simulink model "PEMFuelCellSystem_Cathode_cEGR_SelfHumidifying_v01"  (R2025b)
settings: Solver=VariableStepAuto  StartTime=0.0  StopTime=100  MaxStep=0.1  RelTol=1e-3  AbsTol=1e-3
model workspace (MAT data in the model file):
  Gas_properties_block = 'PEMFuelCellSystem_Before_v01/Anode_Hydrogen_BOP/Gas Mixture
Properties'
  Gas_properties_candidates : object (value not decoded)
  T_TLU = [223.15 228.15 233.15 238.15 243.15 248.15 253.15 258.15 263.15 268.15 272.66 273.15 ... (115 elements, 1x115)]
  air_control_min_current_A = 3.8
  anode_separator_D = 0.02
  anode_separator_T0 = 20
  anode_separator_area = 0.000314159265359
  anode_separator_dp_nominal = 0.0005
  anode_separator_extra_length = 0.04
  anode_separator_laminar_fraction = 0.001
  anode_separator_length = 0.12
  anode_separator_mdot_nominal = 0.01
  anode_separator_p0 = 0.101325
  anode_separator_roughness = 1.5e-05
  anode_tube_D = 0.02
  cathode_channel_dp_nominal_MPa = 0.0368422
  cathode_channel_flow_area_m2 = 0.00403764556423
  cathode_channel_mdot_nominal_kg_s = 0.27182
  cathode_outlet_chamber_V = 0.2
  cathode_separator_D = 0.05
  cathode_separator_T0 = 20
  cathode_separator_area = 0.00407150407905
  cathode_separator_dp_nominal = 0.002
  cathode_separator_extra_length = 0.05
  cathode_separator_laminar_fraction = 0.001
  cathode_separator_length = 0.15
  cathode_separator_mdot_nominal = 0.40798
  cathode_separator_p0 = 0.101325
  cathode_separator_roughness = 1.5e-05
  cathode_tube_D = 0.05
  cegr_comp_map_t_denom_epsilon = 1e-09
  cegr_cond_tau = 1
  cegr_inlet_mixer_p0 = 0.101325
  cegr_outlet_chamber_p0 = 0.101325
  cegr_pipe_D = 0.072
  cegr_pipe_area = 0.00407150407905
  cegr_pipe_extra_length = 0.1
  cegr_pipe_length = 0.5
  cegr_pipe_p0 = 0.101325
  cegr_pipe_roughness = 1.5e-05
  cegr_valve_max_area = 0.001
  cegr_valve_open_min_area = 1e-10
  common_bp_valve_max_area = 0.00134
  common_bp_valve_open_min_area = 1e-10
  comp_inlet_mixer_V = 0.1
  comp_mdot_corr_TLU = [0 0 0 0 0 0.28 0.26 0.24 0.22 0.2 0.56 0.52 ... (15 elements, 5x3)]
  comp_p_ratio_TLU = [1 1.5 2 2.5 3]
  comp_rpm_TLU = [0 50000 80000]
  coolant_num_layers = 20
  coolant_num_passes = 12
  coolant_tube_D = 0.05
  coolant_w_channels = 1
  drive_cycle_current = [0 0 100 100]
  drive_cycle_power = [0 0 40 40]
  drive_cycle_time = [0 0.5 60.5 600]
  drive_cycle_voltage = [427.6 427.6 410 410]
  env_RH = 0.5
  env_T = 20
  env_p = 0.101325
  env_pSat_H2O = 0.00233931818334
  env_yH20 = 0.0115436377169
  env_yO2 = 0.21
  focused_anode_boundary_T_C = 20
  focused_anode_feed_p_MPa_abs = 0.3
  focused_anode_inlet_mdot_kg_s = 0.008
  focused_anode_inlet_p_MPa_abs = 0.161325
  focused_anode_outlet_p_MPa_abs = 0.101325
  focused_anode_pipe_area = 0.00246300864041
  focused_anode_pipe_extra_length = 0.1
  focused_anode_pipe_length = 1
  focused_anode_pipe_roughness = 1.5e-05
  focused_anode_yH2 = 0.9997
  focused_stack_temperature_C = 80
  humidifier_bypass_mode : string (value not decoded)
  intercooler_Dh = 0.05
  intercooler_T0 = 20
  intercooler_area = 0.00785398163397
  intercooler_cond_tau = 1
  intercooler_dp_nominal = 0.005
  intercooler_extra_length = 0.05
  intercooler_laminar_fraction = 0.001
  intercooler_length = 0.25
  intercooler_mdot_nominal = 0.40798
  intercooler_p0 = 0.101325
  intercooler_roughness = 1.5e-05
  pSat_H2O_TLU = [0.0039376926592 0.00720321689378 0.0128411282011 0.0223441068076 0.0380050105363 0.0632733889962 0.103238678713 0.165273175188 0.259872929049 0.401739659013 0.586936061043 0.611151401419 ... (115 elements, 1x115)]
  pSat_TLU = [3379.45709837 5023.40410987 1277.63968517 0.0039376926592 3379.45809837 5023.40510987 1277.64068517 0.00720321689378 3379.45909837 5023.40610987 1277.64168517 0.0128411282011 ... (460 elements, 4x115)]
  radiator_H = 0.5
  radiator_L = 1
  radiator_N_fins = 12000
  radiator_N_tubes = 25
  radiator_W = 0.025
  radiator_air_area_fins = 11.5625
  radiator_air_area_primary = 1.223125
  radiator_cp = 910
  radiator_eta_fin = 0.7
  radiator_fin_spacing = 0.002
  radiator_gap_H = 0.0192708333333
  radiator_rho = 2700
  radiator_t_wall = 0.0001
  radiator_tube_H = 0.0015
  radiator_tube_Leq = 2.5
  routeA_air_control_mode_id = 2
  routeA_air_pid_Ki = 0.5
  routeA_air_pid_Kp = 5
  routeA_anode_inlet_pressure_MPa_abs = 0.161325
  routeA_anode_purge_enable = 1
  routeA_anode_purge_off_n2_mole_fraction = 0.1
  routeA_anode_purge_on_n2_mole_fraction = 0.5
  routeA_anode_recirculation_base_command = 0.2
  routeA_anode_recirculation_current_gain_A_inv = 0.00204081632653
  routeA_anode_rh_setpoint = 1
  routeA_backpressure_control_mode_id = 1
  routeA_cathode_humidifier_gain = 1
  routeA_cathode_rh_setpoint = 1
  routeA_cegr_enabled = 1
  routeA_cegr_valve_mode_id = 1
  routeA_command_profile = [0 0.5 60.5 600 0.101325 0.101325 0.101325 0.101325 20 20 20 20 ... (92 elements, 4x23)]
  routeA_command_profile_baseline = [0.101325 20 0.21 0.0115436377169 0.045 3 0.5 0.1613 1 1 0 70 ... (22 elements, 1x22)]
  routeA_command_profile_fields : string (value not decoded)
  routeA_command_profile_schema : string (value not decoded)
  routeA_current_default_ref_A = 28
  routeA_egr_control_Ki_area = 3.92699081699e-05
  routeA_egr_control_Kp_area = 0.000196349540849
  routeA_egr_control_mode_id = 1
  routeA_egr_target_input_mode_id = 1
  routeA_egr_valve_actuator_tau = 0.5
  routeA_egr_valve_area_direct = 3.92699081699e-06
  routeA_external_case_enabled = 0
  routeA_parameter_layer : string (value not decoded)
  routeA_stack_temperature_set_C = 80
  routeA_target_egr_ratio_comp_in = 0.02
  routeA_voltage_current_max_A = 392
  routeA_voltage_current_min_A = 0
  routeA_voltage_default_ref_V = 394.9
  routeA_voltage_pi_Ki = 0.05
  routeA_voltage_pi_Kp = 1
  separator_condensation_enabled = 1
  separator_l2_efficiency = 0.5
  separator_l2_source : string (value not decoded)
  stack_alpha = 0.7
  stack_area = 380
  stack_iL = 2.5
  stack_io = 0.0001
  stack_mea_cp = 870
  stack_mea_rho = 1800
  stack_num_cells = 606
  stack_num_channels = 8
  stack_t_gdl = 250
  stack_t_membrane = 125
  stack_w_channels = 1.16496474502
  tank_T = 20
  tank_V = 120
  tank_p = 70
  tank_yH2 = 0.9997
libraries: FuelCell_lib x44, nesl_utility x32, fl_lib x32, slpidlib x4
(part 2 of 4)

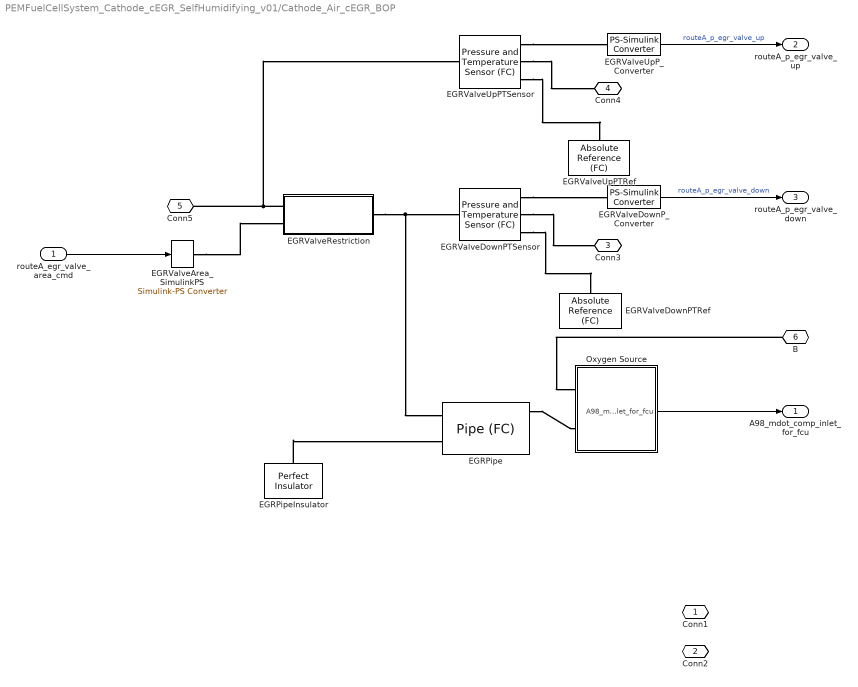
== system PEMFuelCellSystem_Cathode_cEGR_SelfHumidifying_v01/Cathode_Air_cEGR_BOP ==
  routeA_egr_valve_area_cmd : Inport
  EGRPipe : FuelCell_lib/elements/Pipe (FC)  length=cegr_pipe_length m  area=cegr_pipe_area m^2  Dh=cegr_pipe_D m  extra_length=cegr_pipe_extra_length m  roughness=cegr_pipe_roughness m  Re_lam=2000  Re_tur=4000  shape_factor=64  Nu_lam=3.66  tau_c=cegr_cond_tau s  isCond=[0; 0; 0; 1]  volMeas=false  compMeas=FuelCell.enum.Composition.Mole  p0=cegr_pipe_p0 MPa  T0=env_T degC  comp=FuelCell.enum.Composition.Mole  y0=[1-env_yO2-env_yH20; env_yO2; 0; env_yH20]  x0=[1-env_yO2-env_yH20; env_yO2; 0; env_yH20]
      settings: InternalSimscapePortConfiguration="{\"Bottom\":[{\"id\":\"MIn\",\"label\":\"M_in\",\"type\":\"input\"},{\"id\":\"TIn\",\"label\":\"T_in\",\"type\":\"input\"}],\"Left\":[{\"id\":\"A\",\"label\":\"A\",\"type\":\"FuelCell.FuelCell\"},{\"id\":\"H\",\"label\":\"H\",\"type\":\"foundation.thermal.thermal\"}],\"Right\":[{\"id\":\"B\",\"label\":\"B\",\"type\":\"FuelCell.FuelCell\"}],\"Top\":[]}"
  EGRPipeInsulator : fl_lib/Thermal/Thermal Elements/Perfect Insulator  T_specify=off  T_priority=None  T=env_T degC  T_nominal_specify=off  T_nominal_value=1  T_nominal_unit=K
  EGRValveArea_SimulinkPS : nesl_utility/Simulink-PS Converter  PhysicalDomain=network_engine_domain  SubClassName=ps_input  LeftPortType=input  RightPortType=output  PseudoPeriodic=off  Frequencies=[]  NoiseDistribution=none  NoiseParameters=[]  Unit=m^2  AffineConversion=off  FilteringAndDerivatives=provide  SimscapeFilterOrder=1  InputFilterTimeConstant=0.001  UdotUserProvided=0
  EGRValveDownPTRef : FuelCell_lib/elements/Absolute Reference (FC)
      settings: InternalSimscapePortConfiguration="{\"Bottom\":[],\"Left\":[{\"id\":\"A\",\"label\":\"\",\"type\":\"FuelCell.FuelCell\"}],\"Right\":[],\"Top\":[]}"
  EGRValveDownPTSensor : FuelCell_lib/sensors/Pressure and Temperature Sensor (FC)
      settings: InternalSimscapePortConfiguration="{\"Bottom\":[],\"Left\":[{\"id\":\"A\",\"label\":\"A\",\"type\":\"FuelCell.FuelCell\"}],\"Right\":[{\"id\":\"P\",\"label\":\"P\",\"type\":\"output\"},{\"id\":\"T\",\"label\":\"T\",\"type\":\"output\"},{\"id\":\"B\",\"label\":\"B\",\"type\":\"FuelCell.FuelCell\"}],\"Top\":[]}"
  EGRValveDownP_Converter : nesl_utility/PS-Simulink Converter  PhysicalDomain=network_engine_domain  SubClassName=ps_output  LeftPortType=input  RightPortType=output  PseudoPeriodic=off  Frequencies=[]  VectorFormat=inherit  Unit=inherit  AffineConversion=off
  EGRValveRestriction : Subsystem  Variant=on
  EGRValveUpPTRef : FuelCell_lib/elements/Absolute Reference (FC)
      settings: InternalSimscapePortConfiguration="{\"Bottom\":[],\"Left\":[{\"id\":\"A\",\"label\":\"\",\"type\":\"FuelCell.FuelCell\"}],\"Right\":[],\"Top\":[]}"
  EGRValveUpPTSensor : FuelCell_lib/sensors/Pressure and Temperature Sensor (FC)
      settings: InternalSimscapePortConfiguration="{\"Bottom\":[],\"Left\":[{\"id\":\"A\",\"label\":\"A\",\"type\":\"FuelCell.FuelCell\"}],\"Right\":[{\"id\":\"P\",\"label\":\"P\",\"type\":\"output\"},{\"id\":\"T\",\"label\":\"T\",\"type\":\"output\"},{\"id\":\"B\",\"label\":\"B\",\"type\":\"FuelCell.FuelCell\"}],\"Top\":[]}"
  EGRValveUpP_Converter : nesl_utility/PS-Simulink Converter  PhysicalDomain=network_engine_domain  SubClassName=ps_output  LeftPortType=input  RightPortType=output  PseudoPeriodic=off  Frequencies=[]  VectorFormat=inherit  Unit=inherit  AffineConversion=off
  Oxygen Source : Subsystem  Tag=PublishSubsystem
      mask Display:
      | plot(0, 0)
      | plot(100, 100)
      | 
      | n = 80;
      | r1 = 15;
      | r2 = 30;
      | 
      | plot(cos(linspace(0, 2*pi, n))*r1 + 65, sin(linspace(0, 2*pi, n))*r1 + 50)
      | plot(cos(linspace(0, 2*pi, n))*r2 + 65, sin(linspace(0, 2*pi, n))*r2 + 50)
      | 
      | plot([65 30 30 42], [80 80 70 70])
  Conn1 : PMIOPort  Side=Right
  Conn2 : PMIOPort  Port=2  Side=Right
  Conn3 : PMIOPort  Port=3  Side=Right
  Conn4 : PMIOPort  Port=4  Side=Right
  Conn5 : PMIOPort  Port=5  Side=Left
  B : PMIOPort  Port=6  Side=Left
  A98_mdot_comp_inlet_for_fcu : Outport
  routeA_p_egr_valve_up : Outport  Port=2
  routeA_p_egr_valve_down : Outport  Port=3
  wires:
  routeA_egr_valve_area_cmd/1 -> EGRValveArea_SimulinkPS/1
  EGRValveUpP_Converter/1 -> routeA_p_egr_valve_up/1  "routeA_p_egr_valve_up"
  EGRValveDownP_Converter/1 -> routeA_p_egr_valve_down/1  "routeA_p_egr_valve_down"
  Oxygen Source/1(A98_mdot_comp_inlet_for_fcu) -> A98_mdot_comp_inlet_for_fcu/1
  connections:
  EGRValveUpPTSensor/RConn2 -- Conn4/RConn1
  EGRValveUpPTSensor/RConn1 -- EGRValveUpP_Converter/LConn1
  EGRValveArea_SimulinkPS/RConn1 -- EGRValveRestriction/LConn2
  EGRValveRestriction/LConn1 -- Conn5/RConn1 -- EGRValveUpPTSensor/LConn1
  EGRValveRestriction/RConn1 -- EGRPipe/LConn1 -- EGRValveDownPTSensor/LConn1
  EGRPipeInsulator/LConn1 -- EGRPipe/LConn2
  EGRPipe/RConn1 -- Oxygen Source/LConn2
  EGRValveUpPTSensor/RConn3 -- EGRValveUpPTRef/LConn1
  EGRValveDownPTSensor/RConn1 -- EGRValveDownP_Converter/LConn1
  EGRValveDownPTSensor/RConn2 -- Conn3/RConn1
  EGRValveDownPTSensor/RConn3 -- EGRValveDownPTRef/LConn1
  B/RConn1 -- Oxygen Source/LConn1

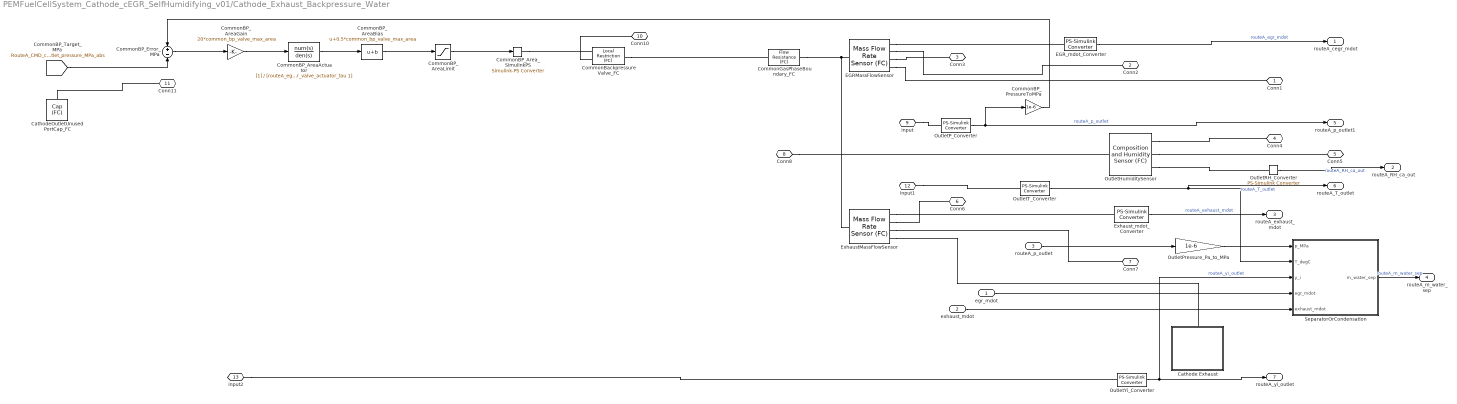
== system PEMFuelCellSystem_Cathode_cEGR_SelfHumidifying_v01/Cathode_Exhaust_Backpressure_Water ==
  egr_mdot : Inport
  exhaust_mdot : Inport  Port=2
  routeA_p_outlet : Inport  Port=3
  Cathode Exhaust : Subsystem  Tag=PublishSubsystem
      settings: PortSchema="{\"entries\":[{\"content\":{\"sides\":[{\"content\":{\"connectorIds\":[]},\"type\":\"ConnectorPlacement.EquallySpacedRectSide\",\"uuid\":\"6344d1cf-22ea-4a51-9588-07afca0fac15\"},{\"content\":{\"connectorIds\":[],\"side\":\"RIGHT\"},\"type\":\"ConnectorPlacement.EquallySpacedRectSide\",\"uuid\":\"a3908f81-9410-4056-87cd-9faba76d3fb8\"},{\"content\":{\"connectorIds\":[\"LConn1\"],\"side\":\"TOP\"},\"type\":\"ConnectorPlacement.EquallySpacedRectSide\",\"uuid\":\"a1c9e24d-adb9-4361-8e9b-feafccbbdb81\"}]},\"type\":\"ConnectorPlacement.EquallySpacedConnector\",\"uuid\":\"d5180d8f-18a0-491d-9fff-909db43c9aea\"}],\"packageUris\":[\"http://schema.mathworks.com/mf0/Connector/R2020b\"],\"version\":\"1.0\"}"
  CathodeOutletUnusedPortCap_FC : FuelCell_lib/elements/Cap (FC)  p_specify=off  p_priority=None  p=101325 Pa  p_nominal_specify=off  p_nominal_value=1  p_nominal_unit=Pa  x_i_specify=off  x_i_priority=None  x_i=[1; 0; 0; 0]  x_i_nominal_specify=off  x_i_nominal_value=1  x_i_nominal_unit=1  T_specify=off  T_priority=None  T=293.15 K  T_nominal_specify=off  T_nominal_value=1  T_nominal_unit=K
      settings: InternalSimscapePortConfiguration="{\"Bottom\":[],\"Left\":[{\"id\":\"A\",\"label\":\"A\",\"type\":\"FuelCell.FuelCell\"}],\"Right\":[],\"Top\":[]}"
  CommonBP_AreaActuator : TransferFcn  Denominator=[routeA_egr_valve_actuator_tau 1]
  CommonBP_AreaBias : Bias  Bias=0.5*common_bp_valve_max_area
  CommonBP_AreaGain : Gain  Gain=20*common_bp_valve_max_area
  CommonBP_AreaLimit : Saturate  UpperLimit=common_bp_valve_max_area  LowerLimit=common_bp_valve_open_min_area
  CommonBP_Area_SimulinkPS : nesl_utility/Simulink-PS Converter  PhysicalDomain=network_engine_domain  SubClassName=ps_input  LeftPortType=input  RightPortType=output  PseudoPeriodic=off  Frequencies=[]  NoiseDistribution=none  NoiseParameters=[]  Unit=m^2  AffineConversion=off  FilteringAndDerivatives=provide  SimscapeFilterOrder=1  InputFilterTimeConstant=0.001  UdotUserProvided=0
  CommonBP_Error_MPa : Sum  Inputs=+-
  CommonBP_PressureToMPa : Gain  Gain=1e-6
  CommonBackpressureValve_FC : FuelCell_lib/elements/Local Restriction (FC)  const_area=false  restriction_area=cegr_valve_area_low m^2  min_area=cegr_valve_open_min_area m^2  max_area=cegr_valve_max_area m^2  area=cegr_pipe_area m^2  Cd=0.64  B_lam=0.999
      settings: InternalSimscapePortConfiguration="{\"Bottom\":[],\"Left\":[{\"id\":\"AR\",\"label\":\"AR\",\"type\":\"input\"},{\"id\":\"A\",\"label\":\"A\",\"type\":\"FuelCell.FuelCell\"}],\"Right\":[{\"id\":\"B\",\"label\":\"B\",\"type\":\"FuelCell.FuelCell\"}],\"Top\":[]}"
  CommonGasPhaseBoundary_FC : FuelCell_lib/elements/Flow Resistance (FC)  var_res=false  delta_p_nominal=cathode_separator_dp_nominal MPa  mdot_nominal=cathode_separator_mdot_nominal kg/s  rho_nominal=0 kg/m^3  laminar_fraction=cathode_separator_laminar_fraction  area=cathode_separator_area m^2  leak_thresh=1e-5
      settings: InternalSimscapePortConfiguration="{\"Bottom\":[],\"Left\":[{\"id\":\"A\",\"label\":\"A\",\"type\":\"FuelCell.FuelCell\"}],\"Right\":[{\"id\":\"B\",\"label\":\"B\",\"type\":\"FuelCell.FuelCell\"}],\"Top\":[]}"
  EGRMassFlowSensor : FuelCell_lib/sensors/Mass Flow Rate Sensor (FC)
      settings: InternalSimscapePortConfiguration="{\"Bottom\":[],\"Left\":[{\"id\":\"A\",\"label\":\"A\",\"type\":\"FuelCell.FuelCell\"}],\"Right\":[{\"id\":\"M\",\"label\":\"M\",\"type\":\"output\"},{\"id\":\"Phi_out\",\"label\":\"Phi\",\"type\":\"output\"},{\"id\":\"M_i\",\"label\":\"M_i\",\"type\":\"output\"},{\"id\":\"B\",\"label\":\"B\",\"type\":\"FuelCell.FuelCell\"}],\"Top\":[]}"
  EGR_mdot_Converter : nesl_utility/PS-Simulink Converter  PhysicalDomain=network_engine_domain  SubClassName=ps_output  LeftPortType=input  RightPortType=output  PseudoPeriodic=off  Frequencies=[]  VectorFormat=inherit  Unit=inherit  AffineConversion=off
  ExhaustMassFlowSensor : FuelCell_lib/sensors/Mass Flow Rate Sensor (FC)
      settings: InternalSimscapePortConfiguration="{\"Bottom\":[],\"Left\":[{\"id\":\"A\",\"label\":\"A\",\"type\":\"FuelCell.FuelCell\"}],\"Right\":[{\"id\":\"M\",\"label\":\"M\",\"type\":\"output\"},{\"id\":\"Phi_out\",\"label\":\"Phi\",\"type\":\"output\"},{\"id\":\"M_i\",\"label\":\"M_i\",\"type\":\"output\"},{\"id\":\"B\",\"label\":\"B\",\"type\":\"FuelCell.FuelCell\"}],\"Top\":[]}"
  Exhaust_mdot_Converter : nesl_utility/PS-Simulink Converter  PhysicalDomain=network_engine_domain  SubClassName=ps_output  LeftPortType=input  RightPortType=output  PseudoPeriodic=off  Frequencies=[]  VectorFormat=inherit  Unit=inherit  AffineConversion=off
  OutletHumiditySensor : FuelCell_lib/sensors/Composition and Humidity Sensor (FC)
      settings: InternalSimscapePortConfiguration="{\"Bottom\":[],\"Left\":[{\"id\":\"A\",\"label\":\"A\",\"type\":\"FuelCell.FuelCell\"}],\"Right\":[{\"id\":\"x_i\",\"label\":\"x_i\",\"type\":\"output\"},{\"id\":\"y_i\",\"label\":\"y_i\",\"type\":\"output\"},{\"id\":\"W\",\"label\":\"W\",\"type\":\"output\"}],\"Top\":[]}"
  OutletP_Converter : nesl_utility/PS-Simulink Converter  PhysicalDomain=network_engine_domain  SubClassName=ps_output  LeftPortType=input  RightPortType=output  PseudoPeriodic=off  Frequencies=[]  VectorFormat=inherit  Unit=inherit  AffineConversion=off
  OutletPressure_Pa_to_MPa : Gain  Gain=1e-6
  OutletRH_Converter : nesl_utility/PS-Simulink Converter  PhysicalDomain=network_engine_domain  SubClassName=ps_output  LeftPortType=input  RightPortType=output  PseudoPeriodic=off  Frequencies=[]  VectorFormat=inherit  Unit=inherit  AffineConversion=off
  OutletT_Converter : nesl_utility/PS-Simulink Converter  PhysicalDomain=network_engine_domain  SubClassName=ps_output  LeftPortType=input  RightPortType=output  PseudoPeriodic=off  Frequencies=[]  VectorFormat=inherit  Unit=inherit  AffineConversion=off
  OutletYi_Converter : nesl_utility/PS-Simulink Converter  PhysicalDomain=network_engine_domain  SubClassName=ps_output  LeftPortType=input  RightPortType=output  PseudoPeriodic=off  Frequencies=[]  VectorFormat=inherit  Unit=inherit  AffineConversion=off
  SeparatorOrCondensation : MATLAB Function  Description=KPI observer only: estimates possible separated or condensed water from outlet p/T/y_i and branch mass flows. It is not the physical separator device.  TreatAsAtomicUnit=on
  Conn1 : PMIOPort  Side=Right
  Conn2 : PMIOPort  Port=2  Side=Right
  Conn3 : PMIOPort  Port=3  Side=Right
  Conn4 : PMIOPort  Port=4  Side=Right
  Conn5 : PMIOPort  Port=5  Side=Right
  Conn6 : PMIOPort  Port=6  Side=Right
  Conn7 : PMIOPort  Port=7  Side=Right
  Conn8 : PMIOPort  Port=8  Side=Left
  input : PMIOPort  Port=9  Side=Left
  Conn10 : PMIOPort  Port=10  Side=Left
  Conn11 : PMIOPort  Port=11  Side=Left
  input1 : PMIOPort  Port=12  Side=Left
  input2 : PMIOPort  Port=13  Side=Left
  routeA_cegr_mdot : Outport
  routeA_RH_ca_out : Outport  Port=2
  routeA_exhaust_mdot : Outport  Port=3
  routeA_m_water_sep : Outport  Port=4
  routeA_p_outlet1 : Outport  Port=5
  routeA_T_outlet : Outport  Port=6
  routeA_yi_outlet : Outport  Port=7
  wires:
  CommonBP_AreaLimit/1 -> CommonBP_Area_SimulinkPS/1
  CommonBP_AreaBias/1 -> CommonBP_AreaLimit/1
  CommonBP_AreaActuator/1 -> CommonBP_AreaBias/1
  CommonBP_AreaGain/1 -> CommonBP_AreaActuator/1
  CommonBP_Error_MPa/1 -> CommonBP_AreaGain/1
  [RouteA_CMD_cathode_outlet_pressure_MPa_abs] -> CommonBP_Error_MPa/2
  CommonBP_PressureToMPa/1 -> CommonBP_Error_MPa/1
  OutletPressure_Pa_to_MPa/1 -> SeparatorOrCondensation/1(p_MPa)
  routeA_p_outlet/1 -> OutletPressure_Pa_to_MPa/1
  OutletRH_Converter/1 -> routeA_RH_ca_out/1  "routeA_RH_ca_out"
  exhaust_mdot/1 -> SeparatorOrCondensation/5(exhaust_mdot)
  OutletYi_Converter/1 -> routeA_yi_outlet/1, SeparatorOrCondensation/3(y_i)  "routeA_yi_outlet"
  SeparatorOrCondensation/1(m_water_sep) -> routeA_m_water_sep/1  "routeA_m_water_sep"
  OutletP_Converter/1 -> CommonBP_PressureToMPa/1, routeA_p_outlet1/1  "routeA_p_outlet"
  EGR_mdot_Converter/1 -> routeA_cegr_mdot/1  "routeA_egr_mdot"
  Exhaust_mdot_Converter/1 -> routeA_exhaust_mdot/1  "routeA_exhaust_mdot"
  OutletT_Converter/1 -> SeparatorOrCondensation/2(T_degC), routeA_T_outlet/1  "routeA_T_outlet"
  egr_mdot/1 -> SeparatorOrCondensation/4(egr_mdot)
  connections:
  CommonBP_Area_SimulinkPS/RConn1 -- CommonBackpressureValve_FC/LConn1
  OutletHumiditySensor/RConn3 -- OutletRH_Converter/LConn1
  OutletHumiditySensor/RConn2 -- Conn5/RConn1
  OutletHumiditySensor/RConn1 -- Conn4/RConn1
  input2/RConn1 -- OutletYi_Converter/LConn1
  ExhaustMassFlowSensor/RConn4 -- Cathode Exhaust/LConn1
  ExhaustMassFlowSensor/RConn3 -- Conn7/RConn1
  ExhaustMassFlowSensor/RConn2 -- Conn6/RConn1
  input/RConn1 -- OutletP_Converter/LConn1
  EGRMassFlowSensor/RConn3 -- Conn3/RConn1
  EGRMassFlowSensor/RConn2 -- Conn2/RConn1
  ExhaustMassFlowSensor/RConn1 -- Exhaust_mdot_Converter/LConn1
  EGRMassFlowSensor/RConn1 -- EGR_mdot_Converter/LConn1
  Conn8/RConn1 -- OutletHumiditySensor/LConn1
  input1/RConn1 -- OutletT_Converter/LConn1
  Conn11/RConn1 -- CathodeOutletUnusedPortCap_FC/LConn1
  EGRMassFlowSensor/LConn1 -- CommonGasPhaseBoundary_FC/RConn1 -- ExhaustMassFlowSensor/LConn1
  EGRMassFlowSensor/RConn4 -- Conn1/RConn1
  Conn10/RConn1 -- CommonBackpressureValve_FC/LConn2
  CommonBackpressureValve_FC/RConn1 -- CommonGasPhaseBoundary_FC/LConn1

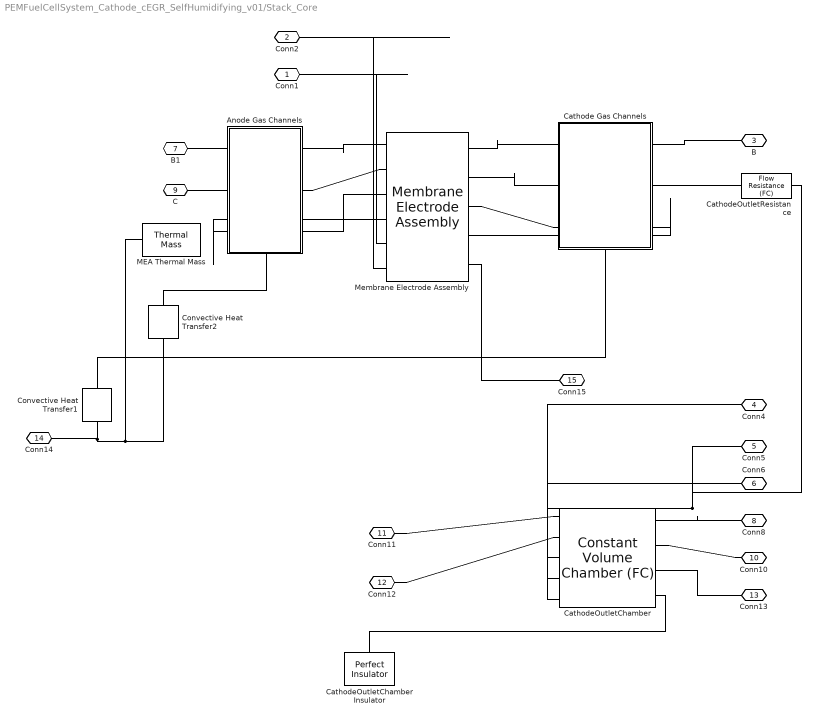
== system PEMFuelCellSystem_Cathode_cEGR_SelfHumidifying_v01/Stack_Core ==
  Anode Gas Channels : Subsystem  Tag=PublishSubsystem
      settings: PortSchema="{\"entries\":[{\"content\":{\"sides\":[{\"content\":{\"connectorIds\":[\"LConn1\",\"LConn2\",\"LConn3\"]},\"type\":\"ConnectorPlacement.EquallySpacedRectSide\",\"uuid\":\"f0c92738-2de1-40ac-9e4a-670524600aa2\"},{\"content\":{\"connectorIds\":[\"RConn1\",\"RConn2\",\"RConn3\"],\"side\":\"RIGHT\"},\"type\":\"ConnectorPlacement.EquallySpacedRectSide\",\"uuid\":\"f0ed995d-2dce-4bd6-9faa-b1cb502a30b1\"},{\"content\":{\"connectorIds\":[],\"side\":\"TOP\"},\"type\":\"ConnectorPlacement.EquallySpacedRectSide\",\"uuid\":\"b5d2d698-46b6-42b5-a767-bb9f1790aa28\"},{\"content\":{\"connectorIds\":[\"RConn4\"],\"side\":\"BOTTOM\"},\"type\":\"ConnectorPlacement.EquallySpacedRectSide\",\"uuid\":\"3e8c99a3-0044-43a9-bacb-b652445e4ac6\"}]},\"type\":\"ConnectorPlacement.EquallySpacedConnector\",\"uuid\":\"912925fb-ca80-4fe6-8a1d-a2308cfd6f88\"}],\"packageUris\":[\"http://schema.mathworks.com/mf0/Connector/R2020b\"],\"version\":\"1.0\"}"
      mask Display:
      | plot(0, 0)
      | plot(100, 100)
      | 
      | x1 = 25;
      | x2 = 65;
      | y1 = 23;
      | y2 = 95;
      | xt = 15;
      | yt = 9;
      | 
      | x_pattern = [x2 x2    x1+xt x1+xt   x1+xt   x2     ];
      | y_pattern = [y2 y2-yt y2-yt y2-2*yt y2-2*yt y2-2*yt];
      | 
      | plot([x1 x1 x2 x_pattern x_pattern      x_pattern      x_pattern         x2    x1], ...
      |      [y1-yt y2 y2 y_pattern y_pattern-2*yt y_pattern-4*yt y_pattern-6*yt y1-yt y1-yt])
  Cathode Gas Channels : Subsystem  Tag=PublishSubsystem
      settings: PortSchema="{\"entries\":[{\"content\":{\"sides\":[{\"content\":{\"connectorIds\":[\"LConn1\",\"LConn2\",\"LConn3\"]},\"type\":\"ConnectorPlacement.EquallySpacedRectSide\",\"uuid\":\"f0c92738-2de1-40ac-9e4a-670524600aa2\"},{\"content\":{\"connectorIds\":[\"RConn1\",\"RConn2\",\"RConn3\"],\"side\":\"RIGHT\"},\"type\":\"ConnectorPlacement.EquallySpacedRectSide\",\"uuid\":\"f0ed995d-2dce-4bd6-9faa-b1cb502a30b1\"},{\"content\":{\"connectorIds\":[],\"side\":\"TOP\"},\"type\":\"ConnectorPlacement.EquallySpacedRectSide\",\"uuid\":\"b5d2d698-46b6-42b5-a767-bb9f1790aa28\"},{\"content\":{\"connectorIds\":[\"RConn4\"],\"side\":\"BOTTOM\"},\"type\":\"ConnectorPlacement.EquallySpacedRectSide\",\"uuid\":\"3e8c99a3-0044-43a9-bacb-b652445e4ac6\"}]},\"type\":\"ConnectorPlacement.EquallySpacedConnector\",\"uuid\":\"912925fb-ca80-4fe6-8a1d-a2308cfd6f88\"}],\"packageUris\":[\"http://schema.mathworks.com/mf0/Connector/R2020b\"],\"version\":\"1.0\"}"
      mask Display:
      | plot(0, 0)
      | plot(100, 100)
      | 
      | x1 = 25;
      | x2 = 65;
      | y1 = 23;
      | y2 = 95;
      | xt = 15;
      | yt = 9;
      | 
      | x_pattern = [x2 x2    x1+xt x1+xt   x1+xt   x2     ];
      | y_pattern = [y2 y2-yt y2-yt y2-2*yt y2-2*yt y2-2*yt];
      | 
      | plot([x1 x1 x2 x_pattern x_pattern      x_pattern      x_pattern         x2    x1], ...
      |      [y1-yt y2 y2 y_pattern y_pattern-2*yt y_pattern-4*yt y_pattern-6*yt y1-yt y1-yt])
  CathodeOutletChamber : FuelCell_lib/elements/Constant Volume Chamber (FC)  V0=cathode_outlet_chamber_V l  num_ports=foundation.enum.num_ports.three  area_A=cegr_pipe_area m^2  area_B=cegr_pipe_area m^2  area_C=cegr_pipe_area m^2  area_D=0.01 m^2  cond_spec=FuelCell.enum.ChamberCondSpec.Enabled  tau_c=cegr_cond_tau s  is_cond=[0; 0; 0; 1]  out_comp=FuelCell.enum.Composition.Mole  p0=cegr_outlet_chamber_p0 MPa  T0=env_T degC  comp=FuelCell.enum.Composition.Mole  y0=[1-env_yO2-env_yH20; env_yO2; 0; env_yH20]  x0=[1-env_yO2-env_yH20; env_yO2; 0; env_yH20]
      settings: InternalSimscapePortConfiguration="{\"Bottom\":[{\"id\":\"H\",\"label\":\"H\",\"type\":\"foundation.thermal.thermal\"}],\"Left\":[{\"id\":\"MIn\",\"label\":\"MIn\",\"type\":\"input\"},{\"id\":\"TIn\",\"label\":\"TIn\",\"type\":\"input\"}],\"Right\":[{\"id\":\"pC\",\"label\":\"p\",\"type\":\"output\"},{\"id\":\"TC\",\"label\":\"T\",\"type\":\"output\"},{\"id\":\"yC_i\",\"label\":\"y_i\",\"type\":\"output\"}],\"Top\":[{\"id\":\"A\",\"label\":\"A\",\"type\":\"FuelCell.FuelCell\"},{\"id\":\"B\",\"label\":\"B\",\"type\":\"FuelCell.FuelCell\"},{\"id\":\"C\",\"label\":\"C\",\"type\":\"FuelCell.FuelCell\"}]}"
  CathodeOutletChamberInsulator : fl_lib/Thermal/Thermal Elements/Perfect Insulator  T_specify=off  T_priority=None  T=env_T degC  T_nominal_specify=off  T_nominal_value=1  T_nominal_unit=K
  CathodeOutletResistance : FuelCell_lib/elements/Flow Resistance (FC)  var_res=false  delta_p_nominal=cathode_channel_dp_nominal_MPa MPa  mdot_nominal=cathode_channel_mdot_nominal_kg_s kg/s  rho_nominal=0 kg/m^3  laminar_fraction=0.1  area=cathode_channel_flow_area_m2 m^2  leak_thresh=1e-5
      settings: InternalSimscapePortConfiguration="{\"Bottom\":[],\"Left\":[{\"id\":\"A\",\"label\":\"A\",\"type\":\"FuelCell.FuelCell\"}],\"Right\":[{\"id\":\"B\",\"label\":\"B\",\"type\":\"FuelCell.FuelCell\"}],\"Top\":[]}"
  Convective Heat Transfer1 : fl_lib/Thermal/Thermal Elements/Convective Heat Transfer  thermal_type=foundation.enum.constant_variable.constant  area=stack_w_channels^2 * stack_num_channels * stack_num_cells cm^2  heat_tr_coeff=10 W/(m^2 * K)  min_heat_tr_coeff=1e-3 W/(K*m^2)  T_specify=off  T_priority=None  T=0 K  T_nominal_specify=off  T_nominal_value=1  T_nominal_unit=K  Q_specify=off  Q_priority=None  Q=0 W  Q_nominal_specify=off  Q_nominal_value=1  Q_nominal_unit=W
  Convective Heat Transfer2 : fl_lib/Thermal/Thermal Elements/Convective Heat Transfer  thermal_type=foundation.enum.constant_variable.constant  area=stack_w_channels^2 * stack_num_channels * stack_num_cells cm^2  heat_tr_coeff=10 W/(m^2 * K)  min_heat_tr_coeff=1e-3 W/(K*m^2)  T_specify=off  T_priority=None  T=0 K  T_nominal_specify=off  T_nominal_value=1  T_nominal_unit=K  Q_specify=off  Q_priority=None  Q=0 W  Q_nominal_specify=off  Q_nominal_value=1  Q_nominal_unit=W
  MEA Thermal Mass : fl_lib/Thermal/Thermal Elements/Thermal Mass  mass_type=foundation.enum.constant_variable.constant  mass=stack_mea_rho * stack_area*1e-4 * (stack_t_membrane + 2*stack_t_gdl)*1e-6 * stack_num_cells kg  sp_heat=stack_mea_cp J/kg/K  mass_min=1e-6 kg  num_ports=foundation.enum.numPorts2.one  m_specify=off  m_priority=High  m=1 kg  m_nominal_specify=off  m_nominal_value=1  m_nominal_unit=kg  T_specify=on  T_priority=High  T=focused_stack_temperature_C degC  T_nominal_specify=off  T_nominal_value=1  T_nominal_unit=K  Q_specify=off  Q_priority=None  Q=0 W  Q_nominal_specify=off  Q_nominal_value=1  Q_nominal_unit=W
  Membrane Electrode Assembly : FuelCell_lib/elements/Membrane Electrode Assembly  N_cell=stack_num_cells  area_cell=stack_area cm^2  t_membrane=stack_t_membrane um  rtype=FuelCell.enum.ResistanceModel.Tabulated1D  RH_TLU=[0, .1, .2, .3, .4, .5, .6, .7, .8, .9, 1]  conductivity_TLU_1D=[0, .017, .035, .055, .081, .11, .15, .21, .27, .35, .45] S/cm  T_scale=1268 K  T_cond=353.15 K  T_TLU=[303.15, 353.15, 393.15] K  conductivity_TLU_2D=[0, .0093, .019, .031, .045, .063, .086, .11, .15, .2, .25; 0, .017, .035, .055, .081, .11, .15, .21, .27, .35, .45; 0, .024, .05, .08, .12, .16, .22, .3, .39, .51, .65] S/cm  io=stack_io A/cm^2  iL=stack_iL A/cm^2  alpha=stack_alpha  rho_membrane=2000 kg/m^3  M_membrane=1.1 kg/mol  D_N2=1e-5 cm^2/s  Icell_specify=off  Icell_priority=None  Icell=0 A  Icell_nominal_specify=off  Icell_nominal_value=1  Icell_nominal_unit=A  HeatRxn_specify=off  HeatRxn_priority=None  HeatRxn=0 W  HeatRxn_nominal_specify=off  HeatRxn_nominal_value=1  HeatRxn_nominal_unit=W  T_stack_specify=off  T_stack_priority=None  T_stack=353.15 K  T_stack_nominal_specify=off  T_stack_nominal_value=1  T_stack_nominal_unit=K
      settings: InternalSimscapePortConfiguration="{\"Bottom\":[{\"id\":\"H\",\"label\":\"H\",\"type\":\"foundation.thermal.thermal\"}],\"Left\":[{\"id\":\"A\",\"label\":\"A\",\"type\":\"FuelCell.FuelCell\"},{\"id\":\"mdot_an\",\"label\":\"Ma\",\"type\":\"output\"},{\"id\":\"T_an\",\"label\":\"Ta\",\"type\":\"output\"},{\"id\":\"x_i_anode\",\"label\":\"xia\",\"type\":\"input\"}],\"Right\":[{\"id\":\"C\",\"label\":\"C\",\"type\":\"FuelCell.FuelCell\"},{\"id\":\"mdot_ca\",\"label\":\"Mc\",\"type\":\"output\"},{\"id\":\"T_ca\",\"label\":\"Tc\",\"type\":\"output\"},{\"id\":\"x_i_cathode\",\"label\":\"xic\",\"type\":\"input\"}],\"Top\":[{\"id\":\"n\",\"label\":\"-\",\"type\":\"foundation.electrical.electrical\"},{\"id\":\"p\",\"label\":\"+\",\"type\":\"foundation.electrical.electrical\"}]}"
  Conn1 : PMIOPort  Side=Left
  Conn2 : PMIOPort  Port=2  Side=Left
  B : PMIOPort  Port=3  Side=Left
  Conn4 : PMIOPort  Port=4  Side=Left
  Conn5 : PMIOPort  Port=5  Side=Right
  Conn6 : PMIOPort  Port=6  Side=Left
  B1 : PMIOPort  Port=7  Side=Left
  Conn8 : PMIOPort  Port=8  Side=Right
  C : PMIOPort  Port=9  Side=Left
  Conn10 : PMIOPort  Port=10  Side=Right
  Conn11 : PMIOPort  Port=11  Side=Left
  Conn12 : PMIOPort  Port=12  Side=Left
  Conn13 : PMIOPort  Port=13  Side=Right
  Conn14 : PMIOPort  Port=14  Side=Left
  Conn15 : PMIOPort  Port=15  Side=Right
  connections:
  CathodeOutletChamberInsulator/LConn1 -- CathodeOutletChamber/RConn4
  Convective Heat Transfer2/LConn1 -- Anode Gas Channels/RConn4
  Convective Heat Transfer1/RConn1 -- Convective Heat Transfer2/RConn1 -- MEA Thermal Mass/LConn1 -- Conn14/RConn1
  Convective Heat Transfer1/LConn1 -- Cathode Gas Channels/RConn4
  C/RConn1 -- Anode Gas Channels/LConn2
  Conn1/RConn1 -- Membrane Electrode Assembly/LConn5
  Membrane Electrode Assembly/RConn1 -- Cathode Gas Channels/RConn1
  Conn2/RConn1 -- Membrane Electrode Assembly/LConn6
  Conn11/RConn1 -- CathodeOutletChamber/LConn1
  B1/RConn1 -- Anode Gas Channels/LConn1
  Anode Gas Channels/LConn3 -- Membrane Electrode Assembly/LConn4
  Anode Gas Channels/RConn1 -- Membrane Electrode Assembly/LConn1
  Anode Gas Channels/RConn2 -- Membrane Electrode Assembly/LConn2
  Anode Gas Channels/RConn3 -- Membrane Electrode Assembly/LConn3
  Membrane Electrode Assembly/RConn5 -- Conn15/RConn1
  Membrane Electrode Assembly/RConn2 -- Cathode Gas Channels/RConn2
  Membrane Electrode Assembly/RConn3 -- Cathode Gas Channels/RConn3
  Membrane Electrode Assembly/RConn4 -- Cathode Gas Channels/LConn3
  Conn12/RConn1 -- CathodeOutletChamber/LConn2
  Cathode Gas Channels/LConn1 -- B/RConn1
  Cathode Gas Channels/LConn2 -- CathodeOutletResistance/LConn1
  CathodeOutletChamber/RConn1 -- Conn8/RConn1
  CathodeOutletChamber/RConn2 -- Conn10/RConn1
  CathodeOutletChamber/RConn3 -- Conn13/RConn1
  CathodeOutletChamber/LConn3 -- Conn5/RConn1 -- CathodeOutletResistance/RConn1
  CathodeOutletChamber/LConn4 -- Conn6/RConn1
  CathodeOutletChamber/LConn5 -- Conn4/RConn1

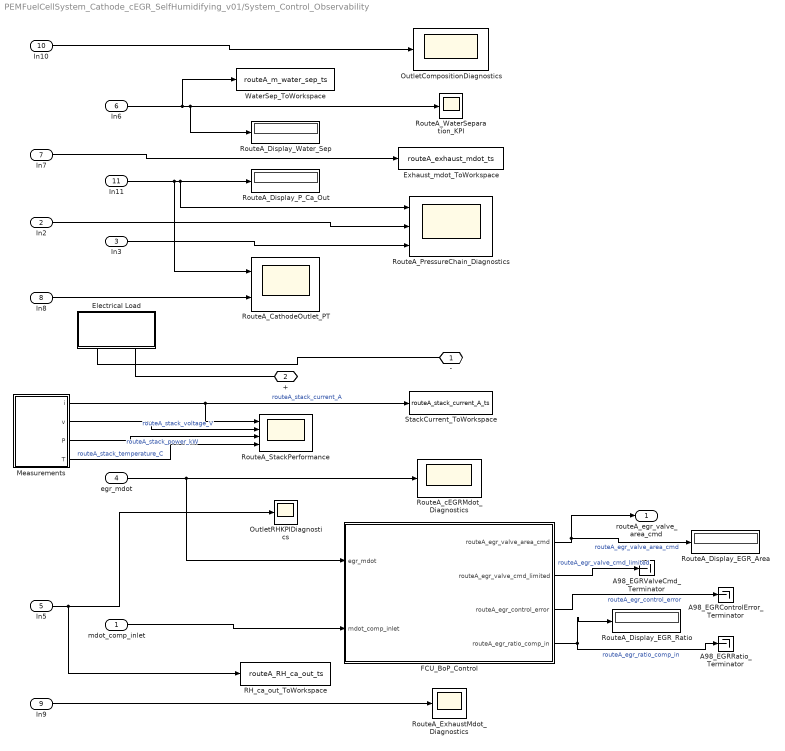
== system PEMFuelCellSystem_Cathode_cEGR_SelfHumidifying_v01/System_Control_Observability ==
  mdot_comp_inlet : Inport
  In2 : Inport  Port=2
  In3 : Inport  Port=3
  egr_mdot : Inport  Port=4
  In5 : Inport  Port=5
  In6 : Inport  Port=6
  In7 : Inport  Port=7
  In8 : Inport  Port=8
  In9 : Inport  Port=9
  In10 : Inport  Port=10
  In11 : Inport  Port=11
  A98_EGRControlError_Terminator : Terminator
  A98_EGRRatio_Terminator : Terminator
  A98_EGRValveCmd_Terminator : Terminator
  Electrical Load : Subsystem  Tag=PublishSubsystem  mask(Electrical Load){input_type=Voltage}
      mask prompts: input_type "Select one of the following scenarios:"
      mask help: Electrical boundary mode selector. input_type activates one demand variant inside Inputs: Current (I_cmd direct), Power (P_cmd -> I_cmd), or Voltage (V_cmd -> PI -> I_cmd). One mode per run; set per-case via SimulationInput.setBlockParameter(...,'input_type',...).
      settings: PortSchema="{\"entries\":[{\"content\":{\"sides\":[{\"content\":{\"connectorIds\":[]},\"type\":\"ConnectorPlacement.EquallySpacedRectSide\",\"uuid\":\"cf26c57a-4aaa-4eca-a1cf-dab3379228b7\"},{\"content\":{\"connectorIds\":[],\"side\":\"RIGHT\"},\"type\":\"ConnectorPlacement.EquallySpacedRectSide\",\"uuid\":\"bd4a28c6-f8d3-4492-9f61-a12eb17ccdd3\"},{\"content\":{\"connectorIds\":[],\"side\":\"TOP\"},\"type\":\"ConnectorPlacement.EquallySpacedRectSide\",\"uuid\":\"7f54a4db-ccf4-4e3a-a135-4ada067d241f\"},{\"content\":{\"connectorIds\":[\"RConn1\",\"RConn2\"],\"side\":\"BOTTOM\"},\"type\":\"ConnectorPlacement.EquallySpacedRectSide\",\"uuid\":\"8817983d-3f79-43b3-9594-6d12f7dcf066\"}]},\"type\":\"ConnectorPlacement.EquallySpacedConnector\",\"uuid\":\"79253ea6-cd7f-4983-840a-f5cee3a4dd91\"}],\"packageUris\":[\"http://schema.mathworks.com/mf0/Connector/R2020b\"],\"version\":\"1.0\"}"
      mask TypeOptions input_type: Current | Power | Voltage
      mask Callback input_type:
      | activeVariant = get_param(gcb, 'input_type');
      | set_param([gcb '/Inputs'], 'OverrideUsingVariant', activeVariant)
      mask Display:
      | blk = get_param([gcb, '/Inputs'], 'CompiledActiveChoiceBlock');
      | eval(get_param(blk, 'MaskDisplay'))
  Exhaust_mdot_ToWorkspace : ToWorkspace  VariableName=routeA_exhaust_mdot_ts  SaveFormat=Timeseries  SampleTime=-1
  FCU_BoP_Control : Subsystem
  Measurements : Subsystem
  OutletCompositionDiagnostics : Scope
  OutletRHKPIDiagnostics : Scope
  RH_ca_out_ToWorkspace : ToWorkspace  VariableName=routeA_RH_ca_out_ts  SaveFormat=Timeseries
  RouteA_CathodeOutlet_PT : Scope  NumInputPorts=2
  RouteA_Display_EGR_Area : Display
  RouteA_Display_EGR_Ratio : Display
  RouteA_Display_P_Ca_Out : Display
  RouteA_Display_Water_Sep : Display
  RouteA_ExhaustMdot_Diagnostics : Scope
  RouteA_PressureChain_Diagnostics : Scope  NumInputPorts=3
  RouteA_StackPerformance : Scope  NumInputPorts=4
      settings: Title=Current (A)  ActiveDisplayYMinimum=-30.6721  ActiveDisplayYMaximum=276.0489
  RouteA_WaterSeparation_KPI : Scope
  RouteA_cEGRMdot_Diagnostics : Scope
  StackCurrent_ToWorkspace : ToWorkspace  VariableName=routeA_stack_current_A_ts  SaveFormat=Timeseries
  WaterSep_ToWorkspace : ToWorkspace  VariableName=routeA_m_water_sep_ts  SaveFormat=Timeseries
  - : PMIOPort  Side=Right
  + : PMIOPort  Port=2  Side=Right
  routeA_egr_valve_area_cmd : Outport
  wires:
  FCU_BoP_Control/1(routeA_egr_valve_area_cmd) -> RouteA_Display_EGR_Area/1, routeA_egr_valve_area_cmd/1  "routeA_egr_valve_area_cmd"
  FCU_BoP_Control/2(routeA_egr_valve_cmd_limited) -> A98_EGRValveCmd_Terminator/1  "routeA_egr_valve_cmd_limited"
  FCU_BoP_Control/3(routeA_egr_control_error) -> A98_EGRControlError_Terminator/1  "routeA_egr_control_error"
  FCU_BoP_Control/4(routeA_egr_ratio_comp_in) -> RouteA_Display_EGR_Ratio/1, A98_EGRRatio_Terminator/1  "routeA_egr_ratio_comp_in"
  In9/1 -> RouteA_ExhaustMdot_Diagnostics/1
  mdot_comp_inlet/1 -> FCU_BoP_Control/2(mdot_comp_inlet)
  Measurements/1(i) -> StackCurrent_ToWorkspace/1, RouteA_StackPerformance/1  "routeA_stack_current_A"
  In8/1 -> RouteA_CathodeOutlet_PT/2
  egr_mdot/1 -> RouteA_cEGRMdot_Diagnostics/1, FCU_BoP_Control/1(egr_mdot)
  In5/1 -> OutletRHKPIDiagnostics/1, RH_ca_out_ToWorkspace/1
  In11/1 -> RouteA_PressureChain_Diagnostics/1, RouteA_Display_P_Ca_Out/1, RouteA_CathodeOutlet_PT/1
  In7/1 -> Exhaust_mdot_ToWorkspace/1
  Measurements/2(v) -> RouteA_StackPerformance/2  "routeA_stack_voltage_V"
  Measurements/3(P) -> RouteA_StackPerformance/3  "routeA_stack_power_kW"
  Measurements/4(T) -> RouteA_StackPerformance/4  "routeA_stack_temperature_C"
  In10/1 -> OutletCompositionDiagnostics/1
  In3/1 -> RouteA_PressureChain_Diagnostics/3
  In2/1 -> RouteA_PressureChain_Diagnostics/2
  In6/1 -> RouteA_Display_Water_Sep/1, RouteA_WaterSeparation_KPI/1, WaterSep_ToWorkspace/1
  connections:
  Electrical Load/RConn1 -- -/RConn1
  Electrical Load/RConn2 -- +/RConn1

== system PEMFuelCellSystem_Cathode_cEGR_SelfHumidifying_v01/cEGR_Mode_Selector ==
  note: 1) Add Subsystem or Model blocks as valid variant choices.
      | 2) You cannot connect blocks at this level. At simulation, connectivity is automatically
      | determined, based on the active variant and port name matching.
  noCEGR_Isolation : Subsystem  VariantControl=routeA_cegr_enabled == 0
  withCEGR_PassThrough : Subsystem  VariantControl=routeA_cegr_enabled == 1
  A : PMIOPort  Side=Left
  B : PMIOPort  Port=2  Side=Left

== system PEMFuelCellSystem_Cathode_cEGR_SelfHumidifying_v01/Cathode_Air_cEGR_BOP/EGRValveRestriction ==
  note: 1) Add Subsystem or Model blocks as valid variant choices.
      | 2) You cannot connect blocks at this level. At simulation, connectivity is automatically
      | determined, based on the active variant and port name matching.
  Closed : Subsystem  VariantControl=routeA_cegr_valve_mode_id == 0
  Open : Subsystem  VariantControl=routeA_cegr_valve_mode_id == 1
  A : PMIOPort  Side=Left
  AR : PMIOPort  Port=2  Side=Left
  B : PMIOPort  Port=3  Side=Right

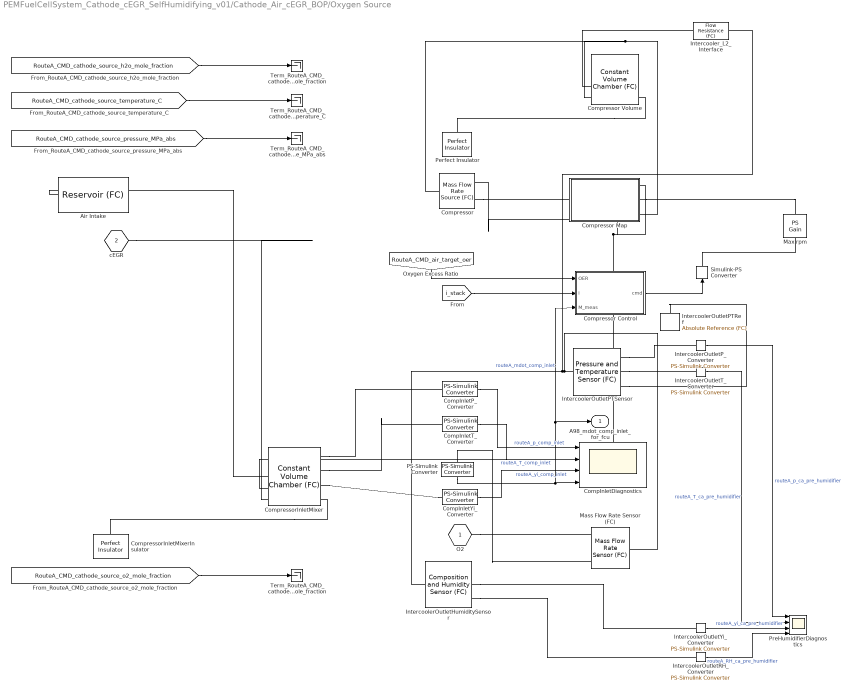
== system PEMFuelCellSystem_Cathode_cEGR_SelfHumidifying_v01/Cathode_Air_cEGR_BOP/Oxygen Source ==
  Air Intake : FuelCell_lib/elements/Reservoir (FC)  constCond=true  p0=env_p MPa  T0=env_T degC  comp=FuelCell.enum.Composition.Mole  y0=[1-env_yO2-env_yH20; env_yO2; 0; env_yH20]  x0=[1; 0; 0; 0]  area=0.01 m^2
      settings: InternalSimscapePortConfiguration="{\"Bottom\":[],\"Left\":[],\"Right\":[],\"Top\":[{\"id\":\"A\",\"label\":\"A\",\"type\":\"FuelCell.FuelCell\"}]}"
  CompInletDiagnostics : Scope  NumInputPorts=4
  CompInletP_Converter : nesl_utility/PS-Simulink Converter  PhysicalDomain=network_engine_domain  SubClassName=ps_output  LeftPortType=input  RightPortType=output  PseudoPeriodic=off  Frequencies=[]  VectorFormat=inherit  Unit=inherit  AffineConversion=off
  CompInletT_Converter : nesl_utility/PS-Simulink Converter  PhysicalDomain=network_engine_domain  SubClassName=ps_output  LeftPortType=input  RightPortType=output  PseudoPeriodic=off  Frequencies=[]  VectorFormat=inherit  Unit=inherit  AffineConversion=off
  CompInletYi_Converter : nesl_utility/PS-Simulink Converter  PhysicalDomain=network_engine_domain  SubClassName=ps_output  LeftPortType=input  RightPortType=output  PseudoPeriodic=off  Frequencies=[]  VectorFormat=inherit  Unit=inherit  AffineConversion=off
  Compressor : FuelCell_lib/sources/Mass Flow Rate Source (FC)  source_type=foundation.enum.constant_controlled.controlled  flow_rate=0 kg/s  power_spec=foundation.enum.power_spec.isentropic  area_A=pi*cathode_tube_D^2/4 m^2  area_B=pi*cathode_tube_D^2/4 m^2  mdot_A_specify=off  mdot_A_priority=None  mdot_A=0.1 kg/s  mdot_A_nominal_specify=off  mdot_A_nominal_value=1  mdot_A_nominal_unit=kg/s  mdot_B_specify=off  mdot_B_priority=None  mdot_B=0.1 kg/s  mdot_B_nominal_specify=off  mdot_B_nominal_value=1  mdot_B_nominal_unit=kg/s  phi_A_specify=off  phi_A_priority=None  phi_A=0 J/s  phi_A_nominal_specify=off  phi_A_nominal_value=1  phi_A_nominal_unit=J/s  phi_B_specify=off  phi_B_priority=None  phi_B=0 J/s  phi_B_nominal_specify=off  phi_B_nominal_value=1  phi_B_nominal_unit=J/s  mdot_A_i_specify=off  mdot_A_i_priority=None  mdot_A_i=[0; 0; 0; 0] kg/s  mdot_A_i_nominal_specify=off  mdot_A_i_nominal_value=1  mdot_A_i_nominal_unit=kg/s  mdot_B_i_specify=off  mdot_B_i_priority=None  mdot_B_i=[0; 0; 0; 0] kg/s  mdot_B_i_nominal_specify=off  mdot_B_i_nominal_value=1  mdot_B_i_nominal_unit=kg/s
      settings: InternalSimscapePortConfiguration="{\"Bottom\":[],\"Left\":[{\"id\":\"M\",\"label\":\"M\",\"type\":\"input\"},{\"id\":\"A\",\"label\":\"A\",\"type\":\"FuelCell.FuelCell\"}],\"Right\":[{\"id\":\"B\",\"label\":\"B\",\"type\":\"FuelCell.FuelCell\"}],\"Top\":[]}"
  Compressor Volume : FuelCell_lib/elements/Constant Volume Chamber (FC)  V0=0.3 l  num_ports=foundation.enum.num_ports.two  area_A=pi*cathode_tube_D^2/4 m^2  area_B=pi*cathode_tube_D^2/4 m^2  area_C=0.01 m^2  area_D=0.01 m^2  cond_spec=FuelCell.enum.ChamberCondSpec.Enabled  tau_c=1e-3 s  is_cond=[0; 0; 0; 0]  out_comp=FuelCell.enum.Composition.Mole  p0=env_p MPa  T0=env_T degC  comp=FuelCell.enum.Composition.Mole  y0=[1-env_yO2-env_yH20; env_yO2; 0; env_yH20]  x0=[1; 0; 0; 0]
      settings: InternalSimscapePortConfiguration="{\"Bottom\":[{\"id\":\"H\",\"label\":\"H\",\"type\":\"foundation.thermal.thermal\"}],\"Left\":[{\"id\":\"MIn\",\"label\":\"MIn\",\"type\":\"input\"},{\"id\":\"TIn\",\"label\":\"TIn\",\"type\":\"input\"}],\"Right\":[{\"id\":\"pC\",\"label\":\"p\",\"type\":\"output\"},{\"id\":\"TC\",\"label\":\"T\",\"type\":\"output\"},{\"id\":\"yC_i\",\"label\":\"y_i\",\"type\":\"output\"}],\"Top\":[{\"id\":\"A\",\"label\":\"A\",\"type\":\"FuelCell.FuelCell\"},{\"id\":\"B\",\"label\":\"B\",\"type\":\"FuelCell.FuelCell\"}]}"
  Compressor Control : Subsystem
  Compressor Map : Subsystem
  CompressorInletMixer : FuelCell_lib/elements/Constant Volume Chamber (FC)  V0=comp_inlet_mixer_V l  num_ports=foundation.enum.num_ports.three  area_A=cegr_pipe_area m^2  area_B=cegr_pipe_area m^2  area_C=cegr_pipe_area m^2  area_D=0.01 m^2  cond_spec=FuelCell.enum.ChamberCondSpec.Enabled  tau_c=cegr_cond_tau s  is_cond=[0; 0; 0; 1]  out_comp=FuelCell.enum.Composition.Mole  p0=cegr_inlet_mixer_p0 MPa  T0=env_T degC  comp=FuelCell.enum.Composition.Mole  y0=[1-env_yO2-env_yH20; env_yO2; 0; env_yH20]  x0=[1; 0; 0; 0]
      settings: InternalSimscapePortConfiguration="{\"Bottom\":[{\"id\":\"H\",\"label\":\"H\",\"type\":\"foundation.thermal.thermal\"}],\"Left\":[{\"id\":\"MIn\",\"label\":\"MIn\",\"type\":\"input\"},{\"id\":\"TIn\",\"label\":\"TIn\",\"type\":\"input\"}],\"Right\":[{\"id\":\"pC\",\"label\":\"p\",\"type\":\"output\"},{\"id\":\"TC\",\"label\":\"T\",\"type\":\"output\"},{\"id\":\"yC_i\",\"label\":\"y_i\",\"type\":\"output\"}],\"Top\":[{\"id\":\"A\",\"label\":\"A\",\"type\":\"FuelCell.FuelCell\"},{\"id\":\"B\",\"label\":\"B\",\"type\":\"FuelCell.FuelCell\"},{\"id\":\"C\",\"label\":\"C\",\"type\":\"FuelCell.FuelCell\"}]}"
  CompressorInletMixerInsulator : fl_lib/Thermal/Thermal Elements/Perfect Insulator  T_specify=off  T_priority=None  T=env_T degC  T_nominal_specify=off  T_nominal_value=1  T_nominal_unit=K
  IntercoolerOutletHumiditySensor : FuelCell_lib/sensors/Composition and Humidity Sensor (FC)
      settings: InternalSimscapePortConfiguration="{\"Bottom\":[],\"Left\":[{\"id\":\"A\",\"label\":\"A\",\"type\":\"FuelCell.FuelCell\"}],\"Right\":[{\"id\":\"x_i\",\"label\":\"x_i\",\"type\":\"output\"},{\"id\":\"y_i\",\"label\":\"y_i\",\"type\":\"output\"},{\"id\":\"W\",\"label\":\"W\",\"type\":\"output\"}],\"Top\":[]}"
  IntercoolerOutletPTRef : FuelCell_lib/elements/Absolute Reference (FC)
      settings: InternalSimscapePortConfiguration="{\"Bottom\":[],\"Left\":[{\"id\":\"A\",\"label\":\"\",\"type\":\"FuelCell.FuelCell\"}],\"Right\":[],\"Top\":[]}"
  IntercoolerOutletPTSensor : FuelCell_lib/sensors/Pressure and Temperature Sensor (FC)
      settings: InternalSimscapePortConfiguration="{\"Bottom\":[],\"Left\":[{\"id\":\"A\",\"label\":\"A\",\"type\":\"FuelCell.FuelCell\"}],\"Right\":[{\"id\":\"P\",\"label\":\"P\",\"type\":\"output\"},{\"id\":\"T\",\"label\":\"T\",\"type\":\"output\"},{\"id\":\"B\",\"label\":\"B\",\"type\":\"FuelCell.FuelCell\"}],\"Top\":[]}"
  IntercoolerOutletP_Converter : nesl_utility/PS-Simulink Converter  PhysicalDomain=network_engine_domain  SubClassName=ps_output  LeftPortType=input  RightPortType=output  PseudoPeriodic=off  Frequencies=[]  VectorFormat=inherit  Unit=inherit  AffineConversion=off
  IntercoolerOutletRH_Converter : nesl_utility/PS-Simulink Converter  PhysicalDomain=network_engine_domain  SubClassName=ps_output  LeftPortType=input  RightPortType=output  PseudoPeriodic=off  Frequencies=[]  VectorFormat=inherit  Unit=inherit  AffineConversion=off
  IntercoolerOutletT_Converter : nesl_utility/PS-Simulink Converter  PhysicalDomain=network_engine_domain  SubClassName=ps_output  LeftPortType=input  RightPortType=output  PseudoPeriodic=off  Frequencies=[]  VectorFormat=inherit  Unit=inherit  AffineConversion=off
  IntercoolerOutletYi_Converter : nesl_utility/PS-Simulink Converter  PhysicalDomain=network_engine_domain  SubClassName=ps_output  LeftPortType=input  RightPortType=output  PseudoPeriodic=off  Frequencies=[]  VectorFormat=inherit  Unit=inherit  AffineConversion=off
  Intercooler_L2_Interface : FuelCell_lib/elements/Flow Resistance (FC)  var_res=false  delta_p_nominal=intercooler_dp_nominal MPa  mdot_nominal=intercooler_mdot_nominal kg/s  rho_nominal=0 kg/m^3  laminar_fraction=intercooler_laminar_fraction  area=intercooler_area m^2  leak_thresh=1e-5
      settings: InternalSimscapePortConfiguration="{\"Bottom\":[],\"Left\":[{\"id\":\"A\",\"label\":\"A\",\"type\":\"FuelCell.FuelCell\"}],\"Right\":[{\"id\":\"B\",\"label\":\"B\",\"type\":\"FuelCell.FuelCell\"}],\"Top\":[]}"
  Mass Flow Rate Sensor (FC) : FuelCell_lib/sensors/Mass Flow Rate Sensor (FC)
      settings: InternalSimscapePortConfiguration="{\"Bottom\":[],\"Left\":[{\"id\":\"A\",\"label\":\"A\",\"type\":\"FuelCell.FuelCell\"}],\"Right\":[{\"id\":\"M\",\"label\":\"M\",\"type\":\"output\"},{\"id\":\"Phi_out\",\"label\":\"Phi\",\"type\":\"output\"},{\"id\":\"M_i\",\"label\":\"M_i\",\"type\":\"output\"},{\"id\":\"B\",\"label\":\"B\",\"type\":\"FuelCell.FuelCell\"}],\"Top\":[]}"
  Max rpm : fl_lib/Physical Signals/Functions/PS Gain  gain=max(comp_rpm_TLU) rpm
  PS-Simulink Converter : nesl_utility/PS-Simulink Converter  PhysicalDomain=network_engine_domain  SubClassName=ps_output  LeftPortType=input  RightPortType=output  PseudoPeriodic=off  Frequencies=[]  VectorFormat=1-D array  Unit=kg/s  AffineConversion=off
  Perfect Insulator : fl_lib/Thermal/Thermal Elements/Perfect Insulator  T_specify=off  T_priority=None  T=env_T degC  T_nominal_specify=off  T_nominal_value=1  T_nominal_unit=K
  PreHumidifierDiagnostics : Scope  NumInputPorts=4
  Simulink-PS Converter : nesl_utility/Simulink-PS Converter  PhysicalDomain=network_engine_domain  SubClassName=ps_input  LeftPortType=input  RightPortType=output  PseudoPeriodic=off  Frequencies=[]  NoiseDistribution=none  NoiseParameters=[]  Unit=1  AffineConversion=off  FilteringAndDerivatives=provide  SimscapeFilterOrder=1  InputFilterTimeConstant=0.001  UdotUserProvided=0
  Term_RouteA_CMD_cathode_source_h2o_mole_fraction : Terminator
  Term_RouteA_CMD_cathode_source_o2_mole_fraction : Terminator
  Term_RouteA_CMD_cathode_source_pressure_MPa_abs : Terminator
  Term_RouteA_CMD_cathode_source_temperature_C : Terminator
  O2 : PMIOPort  Side=Left
  cEGR : PMIOPort  Port=2  Side=Left
  A98_mdot_comp_inlet_for_fcu : Outport
  wires:
  [RouteA_CMD_cathode_source_pressure_MPa_abs] -> Term_RouteA_CMD_cathode_source_pressure_MPa_abs/1
  IntercoolerOutletYi_Converter/1 -> PreHumidifierDiagnostics/3  "routeA_yi_ca_pre_humidifier"
  [i_stack] -> Compressor Control/2(i)
  [RouteA_CMD_cathode_source_temperature_C] -> Term_RouteA_CMD_cathode_source_temperature_C/1
  [RouteA_CMD_cathode_source_h2o_mole_fraction] -> Term_RouteA_CMD_cathode_source_h2o_mole_fraction/1
  [RouteA_CMD_cathode_source_o2_mole_fraction] -> Term_RouteA_CMD_cathode_source_o2_mole_fraction/1
  IntercoolerOutletP_Converter/1 -> PreHumidifierDiagnostics/1  "routeA_p_ca_pre_humidifier"
  CompInletT_Converter/1 -> CompInletDiagnostics/2  "routeA_T_comp_inlet"
  [RouteA_CMD_air_target_oer] -> Compressor Control/1(OER)
  PS-Simulink Converter/1 -> A98_mdot_comp_inlet_for_fcu/1, Compressor Control/3(M_meas), CompInletDiagnostics/4  "routeA_mdot_comp_inlet"
  CompInletP_Converter/1 -> CompInletDiagnostics/1  "routeA_p_comp_inlet"
  IntercoolerOutletT_Converter/1 -> PreHumidifierDiagnostics/2  "routeA_T_ca_pre_humidifier"
  CompInletYi_Converter/1 -> CompInletDiagnostics/3  "routeA_yi_comp_inlet"
  Compressor Control/1(cmd) -> Simulink-PS Converter/1
  IntercoolerOutletRH_Converter/1 -> PreHumidifierDiagnostics/4  "routeA_RH_ca_pre_humidifier"
  connections:
  PS-Simulink Converter/LConn1 -- Mass Flow Rate Sensor (FC)/RConn1
  Compressor/RConn1 -- Compressor Volume/LConn4 -- Compressor Map/RConn3
  IntercoolerOutletHumiditySensor/LConn1 -- IntercoolerOutletPTSensor/LConn1 -- Mass Flow Rate Sensor (FC)/LConn1 -- Intercooler_L2_Interface/RConn1
  CompressorInletMixer/RConn2 -- CompInletT_Converter/LConn1
  IntercoolerOutletPTSensor/RConn3 -- IntercoolerOutletPTRef/LConn1
  Compressor/LConn1 -- Compressor Map/LConn1
  CompressorInletMixerInsulator/LConn1 -- CompressorInletMixer/RConn4
  IntercoolerOutletPTSensor/RConn2 -- IntercoolerOutletT_Converter/LConn1
  Air Intake/LConn1 -- CompressorInletMixer/LConn3
  cEGR/RConn1 -- CompressorInletMixer/LConn5
  CompressorInletMixer/RConn1 -- CompInletP_Converter/LConn1
  CompressorInletMixer/RConn3 -- CompInletYi_Converter/LConn1
  CompressorInletMixer/LConn4 -- Compressor Map/RConn1 -- Compressor/LConn2
  IntercoolerOutletHumiditySensor/RConn2 -- IntercoolerOutletYi_Converter/LConn1
  Perfect Insulator/LConn1 -- Compressor Volume/RConn4
  O2/RConn1 -- Mass Flow Rate Sensor (FC)/RConn4
  IntercoolerOutletHumiditySensor/RConn3 -- IntercoolerOutletRH_Converter/LConn1
  Compressor Volume/LConn3 -- Intercooler_L2_Interface/LConn1
  Compressor Map/RConn2 -- Max rpm/RConn1
  IntercoolerOutletPTSensor/RConn1 -- IntercoolerOutletP_Converter/LConn1
  Simulink-PS Converter/RConn1 -- Max rpm/LConn1
